simulink model "ModeAdjust"  (R2018b)
settings: Solver=FixedStepDiscrete  StartTime=0.0  StopTime=inf  FixedStep=0.01  RelTol=1e-3
undefined symbols (not defined in the file or in its folder): IfKeSMSbSeatMovBkRclnEnable_Val, IfKeSMSbSeatMovFrwdBkwdEnable_Val, IfKeSMSbSeatMovFtrstEnable_Val, IfKeSMSbSeatMovHdrstFrwdBkwdEnable_Val, IfKeSMSbSeatMovHdUpwdDnwdEnable_Val, IfKeSMSbSeatMovLgrstEnable_Val, IfKeSMSbSeatMovLtwdRtwdEnable_Val, IfVeSMSeStNumConfig, KeSMSbArmscreenMovEnable_Val, KeSMSbSeatMovLgrstExpdEnable_Val, KeSMSuFirstRwStBackPosDelta_Val, KeSMSuFirstRwStBackPosTolr_Val, KeSMSuFirstRwStCushFrntPosDelta_Val, KeSMSuFirstRwStCushFrntPosTolr_Val, KeSMSuFirstRwStCushRePosDelta_Val, KeSMSuFirstRwStCushRePosTolr_Val, KeSMSuFirstRwStFootrestPosDelta_Val, KeSMSuFirstRwStFootrestPosTolr_Val, KeSMSuFirstRwStFwdBkwdPosDelta_Val, KeSMSuFirstRwStFwdBkwdPosTolr_Val, KeSMSuMdMotFinshdTm_Val, KeSMSuMdRetryTm1_Val, KeSMSuModeReqDurgTm_Val, KeSMSuSecRwStArmTochPosDelta_Val, KeSMSuSecRwStArmTochPosTolr_Val, KeSMSuSecRwStBackPosDelta_Val, KeSMSuSecRwStBackPosTolr_Val, KeSMSuSecRwStFtrstUpwdDnwdPosDelta_Val, KeSMSuSecRwStFtrstUpwdDnwdPosTolr_Val, KeSMSuSecRwStFwdBkwdPosDelta_Val, KeSMSuSecRwStFwdBkwdPosTolr_Val, KeSMSuSecRwStHeadrestFwdBkwdPosDelta_Val, KeSMSuSecRwStHeadrestFwdBkwdPosTolr_Val, KeSMSuSecRwStHeadrestUpwdDwnwdPosDelta_Val, KeSMSuSecRwStHeadrestUpwdDwnwdPosTolr_Val, KeSMSuSecRwStLegrestInOutPosDelta_Val, KeSMSuSecRwStLegrestInOutPosTolr_Val, KeSMSuSecRwStLegrestUpwdDwnwdPosDelta_Val, KeSMSuSecRwStLegrestUpwdDwnwdPosTolr_Val, KeSMSuSecRwStLwdRwdPosDelta_Val, KeSMSuSecRwStLwdRwdPosTolr_Val, KeSMSuSecRwStVIPFtrstRefAngle_Val, KeSMSuThirdRwStFwdBkwdPosDelta_Val, KeSMSuThirdRwStFwdBkwdPosTolr_Val, KeSMSuThrdRwCushFoldPosDelta_Val, KeSMSuThrdRwCushFoldPosTolr_Val, KeSMSuThrdRwStBackPosDelta_Val, KeSMSuThrdRwStBackPosTolr_Val, KeSMSw4SLegrstCloseMdSecRwLtStFtrstUpwdDnwdPos_Val, KeSMSw4SLegrstCloseMdSecRwLtStFtrstUpwdDnwdPosMax_Val, KeSMSw4SLegrstCloseMdSecRwLtStFtrstUpwdDnwdPosMin_Val, KeSMSw4SLegrstCloseMdSecRwLtStLgrstOtwdInwdPos_Val, KeSMSw4SLegrstCloseMdSecRwLtStLgrstOtwdInwdPosMax_Val, KeSMSw4SLegrstCloseMdSecRwLtStLgrstOtwdInwdPosMin_Val, KeSMSw4SLegrstCloseMdSecRwLtStLgrstUpwdDnwdPos_Val, KeSMSw4SLegrstCloseMdSecRwLtStLgrstUpwdDnwdPosMax_Val, KeSMSw4SLegrstCloseMdSecRwLtStLgrstUpwdDnwdPosMin_Val, KeSMSw4SLegrstCloseMdSecRwRtStFtrstUpwdDnwdPos_Val, KeSMSw4SLegrstCloseMdSecRwRtStFtrstUpwdDnwdPosMax_Val, KeSMSw4SLegrstCloseMdSecRwRtStFtrstUpwdDnwdPosMin_Val ... (+1138)
libraries: Lib x401
(part 34 of 35)

== stateflow chart ModeAdjust/ModeAdjustRunnable_sys/ModeAdjust/OutNumR3_L ==
  (default) -> (junction 87) : {OutNum =0;}
  (junction 87) -> (junction 69) [order 1] : [HaltReq]
  (junction 87) -> (junction 63) [order 2]
  (junction 69) -> (junction 74)
  (junction 63) -> (junction 72) [order 1] : [EZE]
  (junction 63) -> (junction 80) [order 2]
  (junction 72) -> (junction 77) : {OutNum =1;}
  (junction 80) -> (junction 76) [order 1] : [(VIPL&&is6s7s)]
  (junction 80) -> (junction 52) [order 2]
  (junction 76) -> (junction 56) : {OutNum =2;}
  (junction 52) -> (junction 86) [order 1] : [VIPR&&is7s]
  (junction 52) -> (junction 85) [order 2]
  (junction 86) -> (junction 53) : {OutNum =3;}
  (junction 85) -> (junction 90) [order 1] : [Lug]
  (junction 85) -> (junction 81) [order 2]
  (junction 90) -> (junction 59) : {OutNum =4;}
  (junction 81) -> (junction 92) [order 1] : [FAMLY_R]
  (junction 81) -> (junction 97) [order 2]
  (junction 92) -> (junction 94) : {OutNum =5;}
  (junction 97) -> (junction 99) [order 1] : [FAMLY_L]
  (junction 97) -> (junction 104) [order 2]
  (junction 99) -> (junction 101) : {OutNum =6;}
  (junction 101) -> (junction 104)
  (junction 94) -> (junction 101)
  (junction 59) -> (junction 94)
  (junction 53) -> (junction 59)
  (junction 56) -> (junction 53)
  (junction 77) -> (junction 56)
  (junction 74) -> (junction 77)
  data: HaltReq input boolean; EZE input boolean; VIPL input boolean; VIPR input boolean; Lug input boolean; FAMLY_R input boolean; OutNum output uint8; is7s input boolean; is6s7s input boolean; FAMLY_L input boolean

== stateflow chart ModeAdjust/ModeAdjustRunnable_sys/ModeAdjust/OutNumR2_L ==
  (default) -> (junction 115) : {OutNum =0;}
  (junction 115) -> (junction 117) [order 1] : [HaltReq]
  (junction 115) -> (junction 121) [order 2]
  (junction 117) -> (junction 119)
  (junction 121) -> (junction 123) [order 1] : [EZE]
  (junction 121) -> (junction 127) [order 2]
  (junction 123) -> (junction 125) : {OutNum =1;}
  (junction 127) -> (junction 129) [order 1] : [EZQ]
  (junction 127) -> (junction 133) [order 2]
  (junction 129) -> (junction 131) : {OutNum =2;}
  (junction 133) -> (junction 135) [order 1] : [(VIP&&is6s7s)]
  (junction 133) -> (junction 139) [order 2]
  (junction 135) -> (junction 137) : {OutNum =3;}
  (junction 139) -> (junction 141) [order 1] : [(Recovery&&is6s7s)]
  (junction 139) -> (junction 145) [order 2]
  (junction 141) -> (junction 143) : {OutNum =4;}
  (junction 145) -> (junction 147) [order 1] : [INTM]
  (junction 145) -> (junction 151) [order 2]
  (junction 147) -> (junction 149) : {OutNum =5;}
  (junction 151) -> (junction 153) [order 1] : [FAMLY_L]
  (junction 151) -> (junction 157) [order 2]
  (junction 153) -> (junction 155) : {OutNum =6;}
  (junction 157) -> (junction 159) [order 1] : [FAMLY_R]
  (junction 157) -> (junction 164) [order 2]
  (junction 159) -> (junction 161) : {OutNum =7;}
  (junction 164) -> (junction 166) [order 1] : [LyL]
  (junction 164) -> (junction 177) [order 2]
  (junction 166) -> (junction 168) : {OutNum =8;}
  (junction 177) -> (junction 179) [order 1] : [VIP]
  (junction 177) -> (junction 184) [order 2]
  (junction 179) -> (junction 181) : {OutNum =9;}
  (junction 184) -> (junction 186) [order 1] : [Recovery]
  (junction 184) -> (junction 191) [order 2]
  (junction 186) -> (junction 188) : {OutNum =10;}
  (junction 191) -> (junction 193) [order 1] : [INTMR]
  (junction 191) -> (junction 198) [order 2]
  (junction 193) -> (junction 195) : {OutNum =11;}
  (junction 198) -> (junction 200) [order 1] : [LgrstOpen]
  (junction 198) -> (junction 205) [order 2]
  (junction 200) -> (junction 202) : {OutNum =12;}
  (junction 205) -> (junction 207) [order 1] : [LgrstClose]
  (junction 205) -> (junction 212) [order 2]
  (junction 207) -> (junction 209) : {OutNum =13;}
  (junction 209) -> (junction 212)
  (junction 202) -> (junction 209)
  (junction 195) -> (junction 202)
  (junction 188) -> (junction 195)
  (junction 181) -> (junction 188)
  (junction 168) -> (junction 181)
  (junction 161) -> (junction 168)
  (junction 155) -> (junction 161)
  (junction 149) -> (junction 155)
  (junction 143) -> (junction 149)
  (junction 137) -> (junction 143)
  (junction 131) -> (junction 137)
  (junction 125) -> (junction 131)
  (junction 119) -> (junction 125)
  data: HaltReq input boolean; EZE input boolean; EZQ input boolean; VIP input boolean; Recovery input boolean; OutNum output uint8; INTM input boolean; FAMLY_L input boolean; FAMLY_R input boolean; LyL input boolean; is6s7s input boolean; INTMR input boolean; LgrstOpen input boolean; LgrstClose input boolean

== stateflow chart ModeAdjust/ModeAdjustRunnable_sys/ModeAdjust/LyL/Chart ==
  (default) -> (junction 3) : {
      | failflg =0;
      | }
  (junction 3) -> (junction 5) [order 1] : [!R2Lt_ini]
  (junction 5) -> (junction 9) [order 1] : [R2Lt_done]
  (junction 3) -> (junction 13) [order 2] : {R2Lt_En=false;}
  (junction 5) -> (junction 7) [order 2] : {R2Lt_En=true;}
  (junction 9) -> (junction 11) : {R2Lt_En=false;}
  (junction 7) -> (junction 13)
  (junction 11) -> (junction 7)
  (junction 13) -> (junction 183)
  (junction 183) -> (junction 62)
  (junction 62) -> (junction 76) [order 1] : [!Step1_ini]
  (junction 76) -> (junction 64) [order 1] : [pos<openpos1]
  (junction 64) -> (junction 74) [order 1] : [Step1done]
  (junction 62) -> (junction 68) [order 2] : {
      | StepEn_LgrstStep1=false;
      | }
  (junction 76) -> (junction 105) [order 2]
  (junction 64) -> (junction 66) [order 2] : {
      | StepEn_LgrstStep1=true;
      | StepEn_LgrstStep2=false;
      | StepEn_LgrstStep3=false;
      | }
  (junction 74) -> (junction 102) : {
      | StepEn_LgrstStep1=false;
      | StepEn_LgrstStep2=false;
      | StepEn_LgrstStep3=false;
      | failflg =1;
      | }
  (junction 105) -> (junction 107) [order 1] : [!Step2done||Step1done]
  (junction 105) -> (junction 82) [order 2] : {StepEn_LgrstStep1=true;}
  (junction 107) -> (junction 109) : {StepEn_LgrstStep1=false;}
  (junction 82) -> (junction 68)
  (junction 109) -> (junction 82)
  (junction 102) -> (junction 66)
  (junction 68) -> (junction 85)
  (junction 66) -> (junction 99)
  (junction 85) -> (junction 87) [order 1] : [!Step2_ini]
  (junction 87) -> (junction 94) [order 1] : [Step2done]
  (junction 85) -> (junction 89) [order 2] : {
      | StepEn_LgrstStep2=false;
      | }
  (junction 87) -> (junction 91) [order 2] : {
      | StepEn_LgrstStep2=true;
      | }
  (junction 94) -> (junction 96) : {
      | StepEn_LgrstStep2=false;
      | }
  (junction 91) -> (junction 89)
  (junction 96) -> (junction 91)
  (junction 89) -> (junction 101)
  (junction 101) -> (junction 113) [order 1] : [!Step3_ini]
  (junction 113) -> (junction 115) [order 1] : [(!Step2done)||Step3done]
  (junction 101) -> (junction 118) [order 2] : {
      | StepEn_LgrstStep3=false;
      | }
  (junction 113) -> (junction 116) [order 2] : {
      | StepEn_LgrstStep3=true;
      | }
  (junction 115) -> (junction 122) : {
      | StepEn_LgrstStep3=false;
      | }
  (junction 116) -> (junction 118)
  (junction 122) -> (junction 116)
  (junction 99) -> (junction 122)
  (junction 118) -> (junction 125)
  (junction 125) -> (junction 134) [order 1] : [(Step1done&&Step2done&&Step3done)||failflg]
  (junction 134) -> (junction 136) [order 1] : [chkhdflg]
  (junction 136) -> (junction 168) [order 1] : [HdUp_ini||HdUp_Done]
  (junction 168) -> (junction 173) [order 1] : [HdFwd_ini||HdFwd_Done]
  (junction 125) -> (junction 128) [order 2]
  (junction 134) -> (junction 140) [order 2]
  (junction 136) -> (junction 170) [order 2] : {HdUp_En = true;
      | HdFwd_En =false;}
  (junction 168) -> (junction 178) [order 2] : {HdUp_En = false;
      | HdFwd_En =true;}
  (junction 173) -> (junction 175) : {HdUp_En = false;
      | HdFwd_En =false;}
  (junction 140) -> (junction 142) [order 1] : [HdUp_ini||HdUp_Done]
  (junction 140) -> (junction 151) [order 2] : {HdUp_En = true;}
  (junction 142) -> (junction 149) : {HdUp_En =false;}
  (junction 149) -> (junction 151)
  (junction 151) -> (junction 154)
  (junction 154) -> (junction 156) [order 1] : [HdFwd_ini||HdFwd_Done]
  (junction 154) -> (junction 160) [order 2] : {HdFwd_En =true;}
  (junction 156) -> (junction 158) : {HdFwd_En =false;}
  (junction 158) -> (junction 160)
  (junction 160) -> (junction 163)
  (junction 163) -> (junction 128)
  (junction 170) -> (junction 163)
  (junction 178) -> (junction 170)
  (junction 175) -> (junction 178)
  (junction 128) -> (junction 166)
  data: R2Lt_ini input boolean; R2Lt_done input boolean; R2Lt_En output boolean; pos input uint16; openpos1 input uint16; Step1done input boolean; Step2done input boolean; Step3done input boolean; Step1_ini input boolean; Step2_ini input boolean; Step3_ini input boolean; StepEn_LgrstStep1 output boolean; StepEn_LgrstStep2 output boolean; StepEn_LgrstStep3 output boolean; chkhdflg input boolean; HdUp_Done input boolean; HdFwd_Done input boolean; HdUp_En output boolean; HdFwd_En output boolean; failflg output boolean; HdUp_ini input boolean; HdFwd_ini input boolean

== stateflow chart ModeAdjust/ModeAdjustRunnable_sys/ModeAdjust/OutNumR1_L ==
  (default) -> (junction 78) : {OutNum =0;}
  (junction 78) -> (junction 80) [order 1] : [HaltReq||!is6s7s]
  (junction 78) -> (junction 84) [order 2]
  (junction 80) -> (junction 82)
  (junction 84) -> (junction 86) [order 1] : [EZE]
  (junction 84) -> (junction 91) [order 2]
  (junction 86) -> (junction 88) : {OutNum =1;}
  (junction 91) -> (junction 93) [order 1] : [EZQ]
  (junction 91) -> (junction 98) [order 2]
  (junction 93) -> (junction 95) : {OutNum =2;}
  (junction 98) -> (junction 105)
  (junction 105) -> (junction 107) [order 1] : [Recovery_L]
  (junction 105) -> (junction 112) [order 2]
  (junction 107) -> (junction 109) : {OutNum =3;}
  (junction 112) -> (junction 115) [order 1] : [VIP_L]
  (junction 112) -> (junction 117) [order 2]
  (junction 115) -> (junction 119) : {OutNum =4;}
  (junction 119) -> (junction 117)
  (junction 109) -> (junction 119)
  (junction 95) -> (junction 109)
  (junction 88) -> (junction 95)
  (junction 82) -> (junction 88)
  data: HaltReq input boolean; EZE input boolean; EZQ input boolean; OutNum output uint8; Recovery_L input boolean; VIP_L input boolean; is6s7s input boolean

== stateflow chart ModeAdjust/ModeAdjustRunnable_sys/ModeAdjust/OutNumR1_R ==
  (default) -> (junction 115) : {OutNum =0;}
  (junction 115) -> (junction 97) [order 1] : [HaltReq||!is6s7s]
  (junction 115) -> (junction 91) [order 2]
  (junction 97) -> (junction 102)
  (junction 91) -> (junction 100) [order 1] : [EZE]
  (junction 91) -> (junction 108) [order 2]
  (junction 100) -> (junction 105) : {OutNum =1;}
  (junction 108) -> (junction 104) [order 1] : [EZQ]
  (junction 108) -> (junction 90) [order 2]
  (junction 104) -> (junction 84) : {OutNum =2;}
  (junction 90) -> (junction 80)
  (junction 80) -> (junction 114) [order 1] : [Recovery_R]
  (junction 80) -> (junction 113) [order 2]
  (junction 114) -> (junction 81) : {OutNum =3;}
  (junction 113) -> (junction 118) [order 1] : [VIP_R]
  (junction 113) -> (junction 109) [order 2]
  (junction 118) -> (junction 87) : {OutNum =4;}
  (junction 87) -> (junction 109)
  (junction 81) -> (junction 87)
  (junction 84) -> (junction 81)
  (junction 105) -> (junction 84)
  (junction 102) -> (junction 105)
  data: HaltReq input boolean; EZE input boolean; EZQ input boolean; OutNum output uint8; Recovery_R input boolean; VIP_R input boolean; is6s7s input boolean

== stateflow chart ModeAdjust/ModeAdjustRunnable_sys/ModeAdjust/VIPL4s/Chart ==
  (default) -> (junction 3) : {
      | failflg =0;
      | }
  (junction 3) -> (junction 5) [order 1] : [!R2Lt_ini]
  (junction 5) -> (junction 9) [order 1] : [R2Lt_done]
  (junction 3) -> (junction 13) [order 2] : {R2Lt_En=false;}
  (junction 5) -> (junction 7) [order 2] : {R2Lt_En=true;}
  (junction 9) -> (junction 11) : {R2Lt_En=false;}
  (junction 7) -> (junction 13)
  (junction 11) -> (junction 7)
  (junction 13) -> (junction 183)
  (junction 183) -> (junction 62)
  (junction 62) -> (junction 76) [order 1] : [!Step1_ini]
  (junction 76) -> (junction 64) [order 1] : [pos<openpos1]
  (junction 64) -> (junction 74) [order 1] : [Step1done]
  (junction 62) -> (junction 68) [order 2] : {
      | StepEn_LgrstStep1=false;
      | }
  (junction 76) -> (junction 105) [order 2]
  (junction 64) -> (junction 66) [order 2] : {
      | StepEn_LgrstStep1=true;
      | StepEn_LgrstStep2=false;
      | StepEn_LgrstStep3=false;
      | }
  (junction 74) -> (junction 102) : {
      | StepEn_LgrstStep1=false;
      | StepEn_LgrstStep2=false;
      | StepEn_LgrstStep3=false;
      | failflg =1;
      | }
  (junction 105) -> (junction 107) [order 1] : [!Step2done||Step1done]
  (junction 105) -> (junction 82) [order 2] : {StepEn_LgrstStep1=true;}
  (junction 107) -> (junction 109) : {StepEn_LgrstStep1=false;}
  (junction 82) -> (junction 68)
  (junction 109) -> (junction 82)
  (junction 102) -> (junction 66)
  (junction 68) -> (junction 85)
  (junction 66) -> (junction 99)
  (junction 85) -> (junction 87) [order 1] : [!Step2_ini]
  (junction 87) -> (junction 94) [order 1] : [Step2done]
  (junction 85) -> (junction 89) [order 2] : {
      | StepEn_LgrstStep2=false;
      | }
  (junction 87) -> (junction 91) [order 2] : {
      | StepEn_LgrstStep2=true;
      | }
  (junction 94) -> (junction 96) : {
      | StepEn_LgrstStep2=false;
      | }
  (junction 91) -> (junction 89)
  (junction 96) -> (junction 91)
  (junction 89) -> (junction 101)
  (junction 101) -> (junction 113) [order 1] : [!Step3_ini]
  (junction 113) -> (junction 115) [order 1] : [(!Step2done)||Step3done]
  (junction 101) -> (junction 118) [order 2] : {
      | StepEn_LgrstStep3=false;
      | }
  (junction 113) -> (junction 116) [order 2] : {
      | StepEn_LgrstStep3=true;
      | }
  (junction 115) -> (junction 122) : {
      | StepEn_LgrstStep3=false;
      | }
  (junction 116) -> (junction 118)
  (junction 122) -> (junction 116)
  (junction 99) -> (junction 122)
  (junction 118) -> (junction 125)
  (junction 125) -> (junction 134) [order 1] : [(Step1done&&Step2done&&Step3done)||failflg]
  (junction 134) -> (junction 136) [order 1] : [chkhdflg]
  (junction 136) -> (junction 168) [order 1] : [HdUp_ini||HdUp_Done]
  (junction 168) -> (junction 173) [order 1] : [HdFwd_ini||HdFwd_Done]
  (junction 125) -> (junction 128) [order 2]
  (junction 134) -> (junction 140) [order 2]
  (junction 136) -> (junction 170) [order 2] : {HdUp_En = true;
      | HdFwd_En =false;}
  (junction 168) -> (junction 178) [order 2] : {HdUp_En = false;
      | HdFwd_En =true;}
  (junction 173) -> (junction 175) : {HdUp_En = false;
      | HdFwd_En =false;}
  (junction 140) -> (junction 142) [order 1] : [HdUp_ini||HdUp_Done]
  (junction 140) -> (junction 151) [order 2] : {HdUp_En = true;}
  (junction 142) -> (junction 149) : {HdUp_En =false;}
  (junction 149) -> (junction 151)
  (junction 151) -> (junction 154)
  (junction 154) -> (junction 156) [order 1] : [HdFwd_ini||HdFwd_Done]
  (junction 154) -> (junction 160) [order 2] : {HdFwd_En =true;}
  (junction 156) -> (junction 158) : {HdFwd_En =false;}
  (junction 158) -> (junction 160)
  (junction 160) -> (junction 163)
  (junction 163) -> (junction 128)
  (junction 170) -> (junction 163)
  (junction 178) -> (junction 170)
  (junction 175) -> (junction 178)
  (junction 128) -> (junction 166)
  data: R2Lt_ini input boolean; R2Lt_done input boolean; R2Lt_En output boolean; pos input uint16; openpos1 input uint16; Step1done input boolean; Step2done input boolean; Step3done input boolean; Step1_ini input boolean; Step2_ini input boolean; Step3_ini input boolean; StepEn_LgrstStep1 output boolean; StepEn_LgrstStep2 output boolean; StepEn_LgrstStep3 output boolean; chkhdflg input boolean; HdUp_Done input boolean; HdFwd_Done input boolean; HdUp_En output boolean; HdFwd_En output boolean; failflg output boolean; HdUp_ini input boolean; HdFwd_ini input boolean

== stateflow chart ModeAdjust/ModeAdjustRunnable_sys/ModeAdjust/ModeEnChek/Chart3 ==
  (default) -> (junction 3)
  (junction 3) -> (junction 9) : {i = 0;}
  (junction 9) -> (junction 4) [order 1] : [i < 32]
  (junction 4) -> (junction 1) : {
      | temp_var = 0x00000001 & (ModeState32>>i);
      | ModeArray[i] =boolean(temp_var);
      | }
  (junction 1) -> (junction 9) : {i++;}
  (junction 9) -> (junction 5) [order 2]
  data: temp_var local uint32; ModeState32 input uint32; ModeArray output boolean size=32; i local uint8

== stateflow chart ModeAdjust/ModeAdjustRunnable_sys/ModeAdjust/FAMLYL/Chart1 ==
  (default) -> (junction 51)
  (junction 51) -> (junction 53) [order 1] : [LeftDone]
  (junction 51) -> (junction 7) [order 2] : {
      | IfVeSMSbSecRwRtStRclCmdSrv_Val_write=IfVeSMSbSecRwRtStRclCmdSrv_Val_writeRaw;
      | IfVeSMSbThdRwRtStRclCmdSrv_Val_write=IfVeSMSbThdRwRtStRclCmdSrv_Val_writeRaw;
      | IfVeSMSuSecRwLtStRclCmdSrv_Val_write=IfVeSMSuSecRwLtStRclCmdSrv_Val_writeRaw;
      | IfVeSMSbThdRwLtStRclCmdSrv_Val_write=IfVeSMSbThdRwLtStRclCmdSrv_Val_writeRaw;
      | Md_L_DoneOk=false;
      | Md_L_DoneFailed=false;
      | }
  (junction 53) -> (junction 55) : {
      | IfVeSMSbSecRwRtStRclCmdSrv_Val_write=false;
      | IfVeSMSbThdRwRtStRclCmdSrv_Val_write=false;
      | IfVeSMSuSecRwLtStRclCmdSrv_Val_write=false;
      | IfVeSMSbThdRwLtStRclCmdSrv_Val_write=false;
      | Md_L_DoneOk=Md_L_DoneOkRaw;
      | Md_L_DoneFailed=Md_L_DoneFailedRaw;
      | }
  (junction 55) -> (junction 7)
  (junction 7) -> (junction 46)
  data: LeftDone input boolean; IfVeSMSbSecRwRtStRclCmdSrv_Val_write output boolean; IfVeSMSuSecRwLtStRclCmdSrv_Val_write output boolean; IfVeSMSbSecRwRtStRclCmdSrv_Val_writeRaw input; IfVeSMSuSecRwLtStRclCmdSrv_Val_writeRaw input; Md_L_DoneOkRaw input; Md_L_DoneFailedRaw input; Md_L_DoneOk output boolean; Md_L_DoneFailed output boolean; IfVeSMSbThdRwRtStRclCmdSrv_Val_writeRaw input; IfVeSMSbThdRwRtStRclCmdSrv_Val_write output boolean; IfVeSMSbThdRwLtStRclCmdSrv_Val_writeRaw input; IfVeSMSbThdRwLtStRclCmdSrv_Val_write output boolean

== stateflow chart ModeAdjust/ModeAdjustRunnable_sys/ModeAdjust/FAMLYL/Chart2 ==
  (default) -> (junction 487)
  (junction 487) -> (junction 489) [order 1] : [!L_R2Step2_ini]
  (junction 489) -> (junction 488) [order 1] : [L_R2_Step2done]
  (junction 487) -> (junction 483) [order 2] : {L_R2Step2=false;}
  (junction 489) -> (junction 484) [order 2] : {L_R2Step2=true;}
  (junction 488) -> (junction 490) : {L_R2Step2=false;}
  (junction 484) -> (junction 483)
  (junction 490) -> (junction 484)
  (junction 483) -> (junction 460)
  (junction 460) -> (junction 458) [order 1] : [!R_R2Step2_ini]
  (junction 458) -> (junction 463) [order 1] : [R_R2_Step2done]
  (junction 460) -> (junction 466) [order 2] : {R_R2Step2=false;}
  (junction 458) -> (junction 464) [order 2] : {R_R2Step2=true;}
  (junction 463) -> (junction 465) : {R_R2Step2=false;}
  (junction 464) -> (junction 466)
  (junction 465) -> (junction 464)
  (junction 466) -> (junction 461)
  (junction 461) -> (junction 467) [order 1] : [!R_R3_Step1_ini]
  (junction 467) -> (junction 459) [order 1] : [R_R3_Step1done]
  (junction 461) -> (junction 457) [order 2] : {R_R3Step1=false;}
  (junction 467) -> (junction 462) [order 2] : {R_R3Step1=true;}
  (junction 459) -> (junction 455) : {R_R3Step1=false;}
  (junction 462) -> (junction 457)
  (junction 455) -> (junction 462)
  (junction 457) -> (junction 498)
  (junction 498) -> (junction 499) [order 1] : [!L_R3_Step1_ini]
  (junction 499) -> (junction 500) [order 1] : [L_R3_Step1done]
  (junction 498) -> (junction 510) [order 2] : {L_R3Step1=false;}
  (junction 499) -> (junction 508) [order 2] : {L_R3Step1=true;}
  (junction 500) -> (junction 512) : {L_R3Step1=false;}
  (junction 508) -> (junction 510)
  (junction 512) -> (junction 508)
  (junction 510) -> (junction 513)
  data: R_R3Step1 output boolean; R_R2Step2 output boolean; L_R2Step2 output boolean; R_R2Step2_ini input boolean; L_R2Step2_ini input boolean; R_R2_Step2done input boolean; L_R2_Step2done input boolean; R_R3_Step1_ini input boolean; R_R3_Step1done input boolean; L_R3Step1 output boolean; L_R3_Step1_ini input boolean; L_R3_Step1done input boolean

== stateflow chart ModeAdjust/ModeAdjustRunnable_sys/ModeAdjust/FAMLYR/Chart1 ==
  (default) -> (junction 51)
  (junction 51) -> (junction 53) [order 1] : [LeftDone]
  (junction 51) -> (junction 7) [order 2] : {
      | IfVeSMSbSecRwRtStRclCmdSrv_Val_write=IfVeSMSbSecRwRtStRclCmdSrv_Val_writeRaw;
      | IfVeSMSbThdRwRtStRclCmdSrv_Val_write=IfVeSMSbThdRwRtStRclCmdSrv_Val_writeRaw;
      | IfVeSMSuSecRwLtStRclCmdSrv_Val_write=IfVeSMSuSecRwLtStRclCmdSrv_Val_writeRaw;
      | IfVeSMSbThdRwLtStRclCmdSrv_Val_write=IfVeSMSbThdRwLtStRclCmdSrv_Val_writeRaw;
      | Md_L_DoneOk=false;
      | Md_L_DoneFailed=false;
      | }
  (junction 53) -> (junction 55) : {
      | IfVeSMSbSecRwRtStRclCmdSrv_Val_write=false;
      | IfVeSMSbThdRwRtStRclCmdSrv_Val_write=false;
      | IfVeSMSuSecRwLtStRclCmdSrv_Val_write=false;
      | IfVeSMSbThdRwLtStRclCmdSrv_Val_write=false;
      | Md_L_DoneOk=Md_L_DoneOkRaw;
      | Md_L_DoneFailed=Md_L_DoneFailedRaw;
      | }
  (junction 55) -> (junction 7)
  (junction 7) -> (junction 46)
  data: LeftDone input boolean; IfVeSMSbSecRwRtStRclCmdSrv_Val_write output boolean; IfVeSMSuSecRwLtStRclCmdSrv_Val_write output boolean; IfVeSMSbSecRwRtStRclCmdSrv_Val_writeRaw input; IfVeSMSuSecRwLtStRclCmdSrv_Val_writeRaw input; Md_L_DoneOkRaw input; Md_L_DoneFailedRaw input; Md_L_DoneOk output boolean; Md_L_DoneFailed output boolean; IfVeSMSbThdRwRtStRclCmdSrv_Val_writeRaw input; IfVeSMSbThdRwRtStRclCmdSrv_Val_write output boolean; IfVeSMSbThdRwLtStRclCmdSrv_Val_writeRaw input; IfVeSMSbThdRwLtStRclCmdSrv_Val_write output boolean

== stateflow chart ModeAdjust/ModeAdjustRunnable_sys/ModeAdjust/FAMLYR/Chart2 ==
  (default) -> (junction 487)
  (junction 487) -> (junction 489) [order 1] : [!L_R2Step2_ini]
  (junction 489) -> (junction 488) [order 1] : [L_R2_Step2done]
  (junction 487) -> (junction 483) [order 2] : {L_R2Step2=false;}
  (junction 489) -> (junction 484) [order 2] : {L_R2Step2=true;}
  (junction 488) -> (junction 490) : {L_R2Step2=false;}
  (junction 484) -> (junction 483)
  (junction 490) -> (junction 484)
  (junction 483) -> (junction 460)
  (junction 460) -> (junction 458) [order 1] : [!R_R2Step2_ini]
  (junction 458) -> (junction 463) [order 1] : [R_R2_Step2done]
  (junction 460) -> (junction 466) [order 2] : {R_R2Step2=false;}
  (junction 458) -> (junction 464) [order 2] : {R_R2Step2=true;}
  (junction 463) -> (junction 465) : {R_R2Step2=false;}
  (junction 464) -> (junction 466)
  (junction 465) -> (junction 464)
  (junction 466) -> (junction 461)
  (junction 461) -> (junction 467) [order 1] : [!R_R3_Step1_ini]
  (junction 467) -> (junction 459) [order 1] : [R_R3_Step1done]
  (junction 461) -> (junction 457) [order 2] : {R_R3Step1=false;}
  (junction 467) -> (junction 462) [order 2] : {R_R3Step1=true;}
  (junction 459) -> (junction 455) : {R_R3Step1=false;}
  (junction 462) -> (junction 457)
  (junction 455) -> (junction 462)
  (junction 457) -> (junction 511)
  (junction 511) -> (junction 498) [order 1] : [!L_R3_Step1_ini]
  (junction 498) -> (junction 501) [order 1] : [L_R3_Step1done]
  (junction 511) -> (junction 506) [order 2] : {L_R3Step1=false;}
  (junction 498) -> (junction 509) [order 2] : {L_R3Step1=true;}
  (junction 501) -> (junction 505) : {L_R3Step1=false;}
  (junction 509) -> (junction 506)
  (junction 505) -> (junction 509)
  (junction 506) -> (junction 454)
  data: R_R3Step1 output boolean; R_R2Step2 output boolean; L_R2Step2 output boolean; R_R2Step2_ini input boolean; L_R2Step2_ini input boolean; R_R2_Step2done input boolean; L_R2_Step2done input boolean; R_R3_Step1_ini input boolean; R_R3_Step1done input boolean; L_R3Step1 output boolean; L_R3_Step1_ini input boolean; L_R3_Step1done input boolean

== stateflow chart ModeAdjust/ModeAdjustRunnable_sys/ModeAdjust/INTML/Chart ==
  (default) -> (junction 10)
  (junction 10) -> (junction 58) [order 1] : [!L_R2_ini]
  (junction 58) -> (junction 25) [order 1] : [L_R2_done]
  (junction 10) -> (junction 26) [order 2] : {L_R2_en=false;}
  (junction 58) -> (junction 35) [order 2] : {L_R2_en=true;}
  (junction 25) -> (junction 18) : {
      | L_R2_en=false;
      | }
  (junction 35) -> (junction 26)
  (junction 18) -> (junction 35)
  (junction 26) -> (junction 129)
  (junction 129) -> (junction 133) [order 1] : [!R_R2_ini]
  (junction 133) -> (junction 128) [order 1] : [R_R2_done]
  (junction 129) -> (junction 131) [order 2] : {R_R2_en=false;}
  (junction 133) -> (junction 127) [order 2] : {R_R2_en=true;}
  (junction 128) -> (junction 125) : {
      | R_R2_en=false;
      | }
  (junction 127) -> (junction 131)
  (junction 125) -> (junction 127)
  (junction 131) -> (junction 134)
  data: L_R2_ini input boolean; L_R2_done input boolean; R_R2_en output boolean; L_R2_en output boolean; R_R2_ini input boolean; R_R2_done input boolean

== stateflow chart ModeAdjust/ModeAdjustRunnable_sys/ModeAdjust/INTML/Chart1 ==
  (default) -> (junction 1)
  (junction 1) -> (junction 3) [order 1] : [StepAlldone]
  (junction 1) -> (junction 7) [order 2] : {
      | IfVeSMSbSecRwRtStRclCmdSrv_Val_write=IfVeSMSbSecRwRtStRclCmdSrv_Val_writeRaw;
      | IfVeSMSuSecRwLtStRclCmdSrv_Val_write=IfVeSMSuSecRwLtStRclCmdSrv_Val_writeRaw;
      | isINTMDoneOk=false;
      | isINTMDoneFailed=false;
      | }
  (junction 3) -> (junction 5) : {
      | IfVeSMSbSecRwRtStRclCmdSrv_Val_write=false;
      | IfVeSMSuSecRwLtStRclCmdSrv_Val_write=false;
      | isINTMDoneOk=isINTMDoneOkRaw;
      | isINTMDoneFailed=isINTMDoneFailedRaw;
      | }
  (junction 5) -> (junction 7)
  (junction 7) -> (junction 10)
  data: StepAlldone input boolean; IfVeSMSbSecRwRtStRclCmdSrv_Val_write output boolean; IfVeSMSuSecRwLtStRclCmdSrv_Val_write output boolean; isINTMDoneOk output boolean; isINTMDoneFailed output boolean; IfVeSMSbSecRwRtStRclCmdSrv_Val_writeRaw input; IfVeSMSuSecRwLtStRclCmdSrv_Val_writeRaw input; isINTMDoneFailedRaw input; isINTMDoneOkRaw input

== stateflow chart ModeAdjust/ModeAdjustRunnable_sys/ModeAdjust/OutNumR2_R ==
  (default) -> (junction 132) : {OutNum =0;}
  (junction 132) -> (junction 136) [order 1] : [HaltReq]
  (junction 132) -> (junction 134) [order 2]
  (junction 136) -> (junction 183)
  (junction 134) -> (junction 138) [order 1] : [EZE]
  (junction 134) -> (junction 145) [order 2]
  (junction 138) -> (junction 140) : {OutNum =1;}
  (junction 145) -> (junction 147) [order 1] : [EZQ]
  (junction 145) -> (junction 154) [order 2]
  (junction 147) -> (junction 149) : {OutNum =2;}
  (junction 154) -> (junction 156) [order 1] : [(VIP&&is6s7s)]
  (junction 154) -> (junction 163) [order 2]
  (junction 156) -> (junction 158) : {OutNum =3;}
  (junction 163) -> (junction 165) [order 1] : [(Recovery&&is6s7s)]
  (junction 163) -> (junction 172) [order 2]
  (junction 165) -> (junction 167) : {OutNum =4;}
  (junction 172) -> (junction 174) [order 1] : [INTM]
  (junction 172) -> (junction 193) [order 2]
  (junction 174) -> (junction 176) : {OutNum =5;}
  (junction 193) -> (junction 195) [order 1] : [FAMLY_L]
  (junction 193) -> (junction 199) [order 2]
  (junction 195) -> (junction 197) : {OutNum =6;}
  (junction 199) -> (junction 201) [order 1] : [FAMLY_R]
  (junction 199) -> (junction 208) [order 2]
  (junction 201) -> (junction 203) : {OutNum =7;}
  (junction 208) -> (junction 210) [order 1] : [LyR]
  (junction 208) -> (junction 215) [order 2]
  (junction 210) -> (junction 212) : {OutNum =8;}
  (junction 215) -> (junction 217) [order 1] : [VIP]
  (junction 215) -> (junction 223) [order 2]
  (junction 217) -> (junction 219) : {OutNum =9;}
  (junction 223) -> (junction 225) [order 1] : [Recovery]
  (junction 223) -> (junction 230) [order 2]
  (junction 225) -> (junction 227) : {OutNum =10;}
  (junction 230) -> (junction 232) [order 1] : [INTMR]
  (junction 230) -> (junction 237) [order 2]
  (junction 232) -> (junction 234) : {OutNum =11;}
  (junction 237) -> (junction 239) [order 1] : [LgrstOpen]
  (junction 237) -> (junction 244) [order 2]
  (junction 239) -> (junction 241) : {OutNum =12;}
  (junction 244) -> (junction 246) [order 1] : [LgrstClose]
  (junction 244) -> (junction 251) [order 2]
  (junction 246) -> (junction 248) : {OutNum =13;}
  (junction 248) -> (junction 251)
  (junction 241) -> (junction 248)
  (junction 234) -> (junction 241)
  (junction 227) -> (junction 234)
  (junction 219) -> (junction 227)
  (junction 212) -> (junction 219)
  (junction 203) -> (junction 212)
  (junction 197) -> (junction 203)
  (junction 176) -> (junction 197)
  (junction 167) -> (junction 176)
  (junction 158) -> (junction 167)
  (junction 149) -> (junction 158)
  (junction 140) -> (junction 149)
  (junction 183) -> (junction 140)
  data: HaltReq input boolean; EZE input boolean; EZQ input boolean; VIP input boolean; Recovery input boolean; OutNum output uint8; INTM input boolean; FAMLY_L input boolean; FAMLY_R input boolean; LyR input boolean; is6s7s input boolean; INTMR input boolean; LgrstOpen input boolean; LgrstClose input boolean

== stateflow chart ModeAdjust/ModeAdjustRunnable_sys/ModeAdjust/LyL/Chart1 ==
  (default) -> (junction 1)
  (junction 1) -> (junction 3) [order 1] : [Left_Done]
  (junction 1) -> (junction 7) [order 2] : {
      | IfVeSMSuSecRwLtStRclCmdSrv_Val_write=IfVeSMSuSecRwLtStRclCmdSrv_Val_writeRaw;
      | Md_L_DoneOk=false;
      | Md_L_DoneFailed=false;
      | }
  (junction 3) -> (junction 5) : {
      | IfVeSMSuSecRwLtStRclCmdSrv_Val_write=false;
      | Md_L_DoneOk=Md_L_DoneOkRaw;
      | Md_L_DoneFailed=Md_L_DoneFailedRaw;
      | }
  (junction 5) -> (junction 7)
  (junction 7) -> (junction 10)
  data: Left_Done input boolean; IfVeSMSuSecRwLtStRclCmdSrv_Val_write output boolean; IfVeSMSuSecRwLtStRclCmdSrv_Val_writeRaw input; Md_L_DoneOkRaw input; Md_L_DoneFailedRaw input; Md_L_DoneOk output boolean; Md_L_DoneFailed output boolean

== stateflow chart ModeAdjust/ModeAdjustRunnable_sys/ModeAdjust/LyR/Chart ==
  (default) -> (junction 3) : {
      | failflg =0;
      | }
  (junction 3) -> (junction 5) [order 1] : [!R2Lt_ini]
  (junction 5) -> (junction 9) [order 1] : [R2Lt_done]
  (junction 3) -> (junction 13) [order 2] : {R2Lt_En=false;}
  (junction 5) -> (junction 7) [order 2] : {R2Lt_En=true;}
  (junction 9) -> (junction 11) : {R2Lt_En=false;}
  (junction 7) -> (junction 13)
  (junction 11) -> (junction 7)
  (junction 13) -> (junction 183)
  (junction 183) -> (junction 62)
  (junction 62) -> (junction 76) [order 1] : [!Step1_ini]
  (junction 76) -> (junction 64) [order 1] : [pos<openpos1]
  (junction 64) -> (junction 74) [order 1] : [Step1done]
  (junction 62) -> (junction 68) [order 2] : {
      | StepEn_LgrstStep1=false;
      | }
  (junction 76) -> (junction 105) [order 2]
  (junction 64) -> (junction 66) [order 2] : {
      | StepEn_LgrstStep1=true;
      | StepEn_LgrstStep2=false;
      | StepEn_LgrstStep3=false;
      | }
  (junction 74) -> (junction 102) : {
      | StepEn_LgrstStep1=false;
      | StepEn_LgrstStep2=false;
      | StepEn_LgrstStep3=false;
      | failflg =1;
      | }
  (junction 105) -> (junction 107) [order 1] : [!Step2done||Step1done]
  (junction 105) -> (junction 82) [order 2] : {StepEn_LgrstStep1=true;}
  (junction 107) -> (junction 109) : {StepEn_LgrstStep1=false;}
  (junction 82) -> (junction 68)
  (junction 109) -> (junction 82)
  (junction 102) -> (junction 66)
  (junction 68) -> (junction 85)
  (junction 66) -> (junction 99)
  (junction 85) -> (junction 87) [order 1] : [!Step2_ini]
  (junction 87) -> (junction 94) [order 1] : [Step2done]
  (junction 85) -> (junction 89) [order 2] : {
      | StepEn_LgrstStep2=false;
      | }
  (junction 87) -> (junction 91) [order 2] : {
      | StepEn_LgrstStep2=true;
      | }
  (junction 94) -> (junction 96) : {
      | StepEn_LgrstStep2=false;
      | }
  (junction 91) -> (junction 89)
  (junction 96) -> (junction 91)
  (junction 89) -> (junction 101)
  (junction 101) -> (junction 113) [order 1] : [!Step3_ini]
  (junction 113) -> (junction 115) [order 1] : [(!Step2done)||Step3done]
  (junction 101) -> (junction 118) [order 2] : {
      | StepEn_LgrstStep3=false;
      | }
  (junction 113) -> (junction 116) [order 2] : {
      | StepEn_LgrstStep3=true;
      | }
  (junction 115) -> (junction 122) : {
      | StepEn_LgrstStep3=false;
      | }
  (junction 116) -> (junction 118)
  (junction 122) -> (junction 116)
  (junction 99) -> (junction 122)
  (junction 118) -> (junction 125)
  (junction 125) -> (junction 134) [order 1] : [(Step1done&&Step2done&&Step3done)||failflg]
  (junction 134) -> (junction 136) [order 1] : [chkhdflg]
  (junction 136) -> (junction 168) [order 1] : [HdUp_ini||HdUp_Done]
  (junction 168) -> (junction 173) [order 1] : [HdFwd_ini||HdFwd_Done]
  (junction 125) -> (junction 128) [order 2]
  (junction 134) -> (junction 140) [order 2]
  (junction 136) -> (junction 170) [order 2] : {HdUp_En = true;
      | HdFwd_En =false;}
  (junction 168) -> (junction 178) [order 2] : {HdUp_En = false;
      | HdFwd_En =true;}
  (junction 173) -> (junction 175) : {HdUp_En = false;
      | HdFwd_En =false;}
  (junction 140) -> (junction 142) [order 1] : [HdUp_ini||HdUp_Done]
  (junction 140) -> (junction 151) [order 2] : {HdUp_En = true;}
  (junction 142) -> (junction 149) : {HdUp_En =false;}
  (junction 149) -> (junction 151)
  (junction 151) -> (junction 154)
  (junction 154) -> (junction 156) [order 1] : [HdFwd_ini||HdFwd_Done]
  (junction 154) -> (junction 160) [order 2] : {HdFwd_En =true;}
  (junction 156) -> (junction 158) : {HdFwd_En =false;}
  (junction 158) -> (junction 160)
  (junction 160) -> (junction 163)
  (junction 163) -> (junction 128)
  (junction 170) -> (junction 163)
  (junction 178) -> (junction 170)
  (junction 175) -> (junction 178)
  (junction 128) -> (junction 166)
  data: R2Lt_ini input boolean; R2Lt_done input boolean; R2Lt_En output boolean; pos input uint16; openpos1 input uint16; Step1done input boolean; Step2done input boolean; Step3done input boolean; Step1_ini input boolean; Step2_ini input boolean; Step3_ini input boolean; StepEn_LgrstStep1 output boolean; StepEn_LgrstStep2 output boolean; StepEn_LgrstStep3 output boolean; chkhdflg input boolean; HdUp_Done input boolean; HdFwd_Done input boolean; HdUp_En output boolean; HdFwd_En output boolean; failflg output boolean; HdUp_ini input boolean; HdFwd_ini input boolean

== stateflow chart ModeAdjust/ModeAdjustRunnable_sys/ModeAdjust/LyR/Chart1 ==
  (default) -> (junction 1)
  (junction 1) -> (junction 3) [order 1] : [Left_Done]
  (junction 1) -> (junction 7) [order 2] : {
      | IfVeSMSuSecRwLtStRclCmdSrv_Val_write=IfVeSMSuSecRwLtStRclCmdSrv_Val_writeRaw;
      | Md_L_DoneOk=false;
      | Md_L_DoneFailed=false;
      | }
  (junction 3) -> (junction 5) : {
      | IfVeSMSuSecRwLtStRclCmdSrv_Val_write=false;
      | Md_L_DoneOk=Md_L_DoneOkRaw;
      | Md_L_DoneFailed=Md_L_DoneFailedRaw;
      | }
  (junction 5) -> (junction 7)
  (junction 7) -> (junction 10)
  data: Left_Done input boolean; IfVeSMSuSecRwLtStRclCmdSrv_Val_write output boolean; IfVeSMSuSecRwLtStRclCmdSrv_Val_writeRaw input; Md_L_DoneOkRaw input; Md_L_DoneFailedRaw input; Md_L_DoneOk output boolean; Md_L_DoneFailed output boolean

== stateflow chart ModeAdjust/ModeAdjustRunnable_sys/ModeAdjust/VIPR4s/Chart ==
  (default) -> (junction 3) : {
      | failflg =0;
      | }
  (junction 3) -> (junction 5) [order 1] : [!R2Lt_ini]
  (junction 5) -> (junction 9) [order 1] : [R2Lt_done]
  (junction 3) -> (junction 13) [order 2] : {R2Lt_En=false;}
  (junction 5) -> (junction 7) [order 2] : {R2Lt_En=true;}
  (junction 9) -> (junction 11) : {R2Lt_En=false;}
  (junction 7) -> (junction 13)
  (junction 11) -> (junction 7)
  (junction 13) -> (junction 183)
  (junction 183) -> (junction 62)
  (junction 62) -> (junction 76) [order 1] : [!Step1_ini]
  (junction 76) -> (junction 64) [order 1] : [pos<openpos1]
  (junction 64) -> (junction 74) [order 1] : [Step1done]
  (junction 62) -> (junction 68) [order 2] : {
      | StepEn_LgrstStep1=false;
      | }
  (junction 76) -> (junction 105) [order 2]
  (junction 64) -> (junction 66) [order 2] : {
      | StepEn_LgrstStep1=true;
      | StepEn_LgrstStep2=false;
      | StepEn_LgrstStep3=false;
      | }
  (junction 74) -> (junction 102) : {
      | StepEn_LgrstStep1=false;
      | StepEn_LgrstStep2=false;
      | StepEn_LgrstStep3=false;
      | failflg =1;
      | }
  (junction 105) -> (junction 107) [order 1] : [!Step2done||Step1done]
  (junction 105) -> (junction 82) [order 2] : {StepEn_LgrstStep1=true;}
  (junction 107) -> (junction 109) : {StepEn_LgrstStep1=false;}
  (junction 82) -> (junction 68)
  (junction 109) -> (junction 82)
  (junction 102) -> (junction 66)
  (junction 68) -> (junction 85)
  (junction 66) -> (junction 99)
  (junction 85) -> (junction 87) [order 1] : [!Step2_ini]
  (junction 87) -> (junction 94) [order 1] : [Step2done]
  (junction 85) -> (junction 89) [order 2] : {
      | StepEn_LgrstStep2=false;
      | }
  (junction 87) -> (junction 91) [order 2] : {
      | StepEn_LgrstStep2=true;
      | }
  (junction 94) -> (junction 96) : {
      | StepEn_LgrstStep2=false;
      | }
  (junction 91) -> (junction 89)
  (junction 96) -> (junction 91)
  (junction 89) -> (junction 101)
  (junction 101) -> (junction 113) [order 1] : [!Step3_ini]
  (junction 113) -> (junction 115) [order 1] : [(!Step2done)||Step3done]
  (junction 101) -> (junction 118) [order 2] : {
      | StepEn_LgrstStep3=false;
      | }
  (junction 113) -> (junction 116) [order 2] : {
      | StepEn_LgrstStep3=true;
      | }
  (junction 115) -> (junction 122) : {
      | StepEn_LgrstStep3=false;
      | }
  (junction 116) -> (junction 118)
  (junction 122) -> (junction 116)
  (junction 99) -> (junction 122)
  (junction 118) -> (junction 125)
  (junction 125) -> (junction 134) [order 1] : [(Step1done&&Step2done&&Step3done)||failflg]
  (junction 134) -> (junction 136) [order 1] : [chkhdflg]
  (junction 136) -> (junction 168) [order 1] : [HdUp_ini||HdUp_Done]
  (junction 168) -> (junction 173) [order 1] : [HdFwd_ini||HdFwd_Done]
  (junction 125) -> (junction 128) [order 2]
  (junction 134) -> (junction 140) [order 2]
  (junction 136) -> (junction 170) [order 2] : {HdUp_En = true;
      | HdFwd_En =false;}
  (junction 168) -> (junction 178) [order 2] : {HdUp_En = false;
      | HdFwd_En =true;}
  (junction 173) -> (junction 175) : {HdUp_En = false;
      | HdFwd_En =false;}
  (junction 140) -> (junction 142) [order 1] : [HdUp_ini||HdUp_Done]
  (junction 140) -> (junction 151) [order 2] : {HdUp_En = true;}
  (junction 142) -> (junction 149) : {HdUp_En =false;}
  (junction 149) -> (junction 151)
  (junction 151) -> (junction 154)
  (junction 154) -> (junction 156) [order 1] : [HdFwd_ini||HdFwd_Done]
  (junction 154) -> (junction 160) [order 2] : {HdFwd_En =true;}
  (junction 156) -> (junction 158) : {HdFwd_En =false;}
  (junction 158) -> (junction 160)
  (junction 160) -> (junction 163)
  (junction 163) -> (junction 128)
  (junction 170) -> (junction 163)
  (junction 178) -> (junction 170)
  (junction 175) -> (junction 178)
  (junction 128) -> (junction 166)
  data: R2Lt_ini input boolean; R2Lt_done input boolean; R2Lt_En output boolean; pos input uint16; openpos1 input uint16; Step1done input boolean; Step2done input boolean; Step3done input boolean; Step1_ini input boolean; Step2_ini input boolean; Step3_ini input boolean; StepEn_LgrstStep1 output boolean; StepEn_LgrstStep2 output boolean; StepEn_LgrstStep3 output boolean; chkhdflg input boolean; HdUp_Done input boolean; HdFwd_Done input boolean; HdUp_En output boolean; HdFwd_En output boolean; failflg output boolean; HdUp_ini input boolean; HdFwd_ini input boolean

== stateflow chart ModeAdjust/ModeAdjustRunnable_sys/ModeAdjust/VIPL4s/Chart1 ==
  (default) -> (junction 1)
  (junction 1) -> (junction 3) [order 1] : [Left_Done]
  (junction 1) -> (junction 7) [order 2] : {
      | IfVeSMSuSecRwLtStRclCmdSrv_Val_write=IfVeSMSuSecRwLtStRclCmdSrv_Val_writeRaw;
      | Md_L_DoneOk=false;
      | Md_L_DoneFailed=false;
      | }
  (junction 3) -> (junction 5) : {
      | IfVeSMSuSecRwLtStRclCmdSrv_Val_write=false;
      | Md_L_DoneOk=Md_L_DoneOkRaw;
      | Md_L_DoneFailed=Md_L_DoneFailedRaw;
      | }
  (junction 5) -> (junction 7)
  (junction 7) -> (junction 10)
  data: Left_Done input boolean; IfVeSMSuSecRwLtStRclCmdSrv_Val_write output boolean; IfVeSMSuSecRwLtStRclCmdSrv_Val_writeRaw input; Md_L_DoneOkRaw input; Md_L_DoneFailedRaw input; Md_L_DoneOk output boolean; Md_L_DoneFailed output boolean

== stateflow chart ModeAdjust/ModeAdjustRunnable_sys/ModeAdjust/ArrivedAtTargetPosChk/VIP/Pass/FtTargtCal ==
  (default) -> (junction 4)
  (junction 4) -> (junction 6) : {
      | FtTargetAngle = KeSMSuSecRwStVIPFtrstRefAngle-BkReclnUpwdDnwdPos/4000*78;
      | }
  (junction 6) -> (junction 9) [order 1] : [FtTargetAngle<0]
  (junction 6) -> (junction 13) [order 2]
  (junction 9) -> (junction 11) : {
      | FtTargetAngle=0;
      | }
  (junction 11) -> (junction 13)
  (junction 13) -> (junction 16)
  (junction 16) -> (junction 18) [order 1] : [FtTargetAngle>=108.2216]
  (junction 16) -> (junction 25) [order 2] : {
      | n=(sqrt(26933.84-(cos(FtTargetAngle*3.14159/180+0.43)*8110))-139.91)/0.12;
      | }
  (junction 18) -> (junction 20) : {
      | FtTargetPos=4000;
      | }
  (junction 25) -> (junction 28) : {
      | tmpTargetPos = n*4000;
      | tmpTargetPos = tmpTargetPos/335.245;
      | FtTargetPos = tmpTargetPos;
      | }
  (junction 20) -> (junction 28)
  (junction 28) -> (junction 32)
  data: BkReclnUpwdDnwdPos input single; KeSMSuSecRwStVIPFtrstRefAngle input single; FtTargetPos output uint16; FtTargetAngle local single; n local single; tmpTargetPos local single

== stateflow chart ModeAdjust/ModeAdjustRunnable_sys/ModeAdjust/VIPR4s/Chart1 ==
  (default) -> (junction 1)
  (junction 1) -> (junction 3) [order 1] : [Left_Done]
  (junction 1) -> (junction 7) [order 2] : {
      | IfVeSMSuSecRwLtStRclCmdSrv_Val_write=IfVeSMSuSecRwLtStRclCmdSrv_Val_writeRaw;
      | Md_L_DoneOk=false;
      | Md_L_DoneFailed=false;
      | }
  (junction 3) -> (junction 5) : {
      | IfVeSMSuSecRwLtStRclCmdSrv_Val_write=false;
      | Md_L_DoneOk=Md_L_DoneOkRaw;
      | Md_L_DoneFailed=Md_L_DoneFailedRaw;
      | }
  (junction 5) -> (junction 7)
  (junction 7) -> (junction 10)
  data: Left_Done input boolean; IfVeSMSuSecRwLtStRclCmdSrv_Val_write output boolean; IfVeSMSuSecRwLtStRclCmdSrv_Val_writeRaw input; Md_L_DoneOkRaw input; Md_L_DoneFailedRaw input; Md_L_DoneOk output boolean; Md_L_DoneFailed output boolean

== stateflow chart ModeAdjust/ModeAdjustRunnable_sys/ModeAdjust/RecvyL4s/Chart ==
  (default) -> (junction 3) : {failflg=0;}
  (junction 3) -> (junction 5) [order 1] : [!R2Lt_ini]
  (junction 5) -> (junction 9) [order 1] : [R2Lt_done]
  (junction 3) -> (junction 13) [order 2] : {R2Lt_En=false;}
  (junction 5) -> (junction 7) [order 2] : {R2Lt_En=true;}
  (junction 9) -> (junction 11) : {R2Lt_En=false;}
  (junction 7) -> (junction 13)
  (junction 11) -> (junction 7)
  (junction 13) -> (junction 237)
  (junction 237) -> (junction 244) [order 1] : [!HdUp_ini]
  (junction 244) -> (junction 234) [order 1] : [HdUp_Done]
  (junction 237) -> (junction 235) [order 2] : {HdUp_En =false;}
  (junction 244) -> (junction 246) [order 2] : {HdUp_En = true;}
  (junction 234) -> (junction 236) : {HdUp_En =false;}
  (junction 246) -> (junction 235)
  (junction 236) -> (junction 246)
  (junction 235) -> (junction 62)
  (junction 62) -> (junction 105) [order 1] : [!Step1_ini]
  (junction 105) -> (junction 107) [order 1] : [Step1done]
  (junction 62) -> (junction 68) [order 2] : {
      | StepEn_LgrstStep1=false;
      | }
  (junction 105) -> (junction 82) [order 2] : {StepEn_LgrstStep1=true;}
  (junction 107) -> (junction 109) : {StepEn_LgrstStep1=false;}
  (junction 82) -> (junction 68)
  (junction 109) -> (junction 82)
  (junction 68) -> (junction 143)
  (junction 143) -> (junction 142) [order 1] : [!Step2_ini]
  (junction 142) -> (junction 157) [order 1] : [downpos<=closedownpos2&&Ftpos>=FtposDelta]
  (junction 157) -> (junction 224) [order 1] : [Step1done&&Step3done]
  (junction 143) -> (junction 89) [order 2] : {
      | StepEn_LgrstStep2=false;
      | }
  (junction 142) -> (junction 154) [order 2]
  (junction 157) -> (junction 159) [order 2] : {
      | StepEn_LgrstStep2=false;
      | }
  (junction 224) -> (junction 228) : {failflg=1;}
  (junction 154) -> (junction 148) [order 1] : [downpos<closedownpos1&&Otpos>closeOtpos1]
  (junction 154) -> (junction 87) [order 2]
  (junction 148) -> (junction 150) : {StepEn_LgrstStep2 = false;}
  (junction 87) -> (junction 94) [order 1] : [Step2done]
  (junction 87) -> (junction 91) [order 2] : {
      | StepEn_LgrstStep2=true;
      | }
  (junction 94) -> (junction 96) : {
      | StepEn_LgrstStep2=false;
      | }
  (junction 91) -> (junction 89)
  (junction 96) -> (junction 91)
  (junction 150) -> (junction 96)
  (junction 159) -> (junction 150)
  (junction 228) -> (junction 159)
  (junction 89) -> (junction 101)
  (junction 101) -> (junction 113) [order 1] : [!Step3_ini]
  (junction 113) -> (junction 115) [order 1] : [Step3done||!Step1done]
  (junction 101) -> (junction 118) [order 2] : {
      | StepEn_LgrstStep3=false;
      | }
  (junction 113) -> (junction 258) [order 2]
  (junction 115) -> (junction 122) : {
      | StepEn_LgrstStep3=false;
      | }
  (junction 258) -> (junction 260) [order 1] : [downpos>closedownpos2]
  (junction 260) -> (junction 274) [order 1] : [Step2done]
  (junction 258) -> (junction 116) [order 2] : {
      | StepEn_LgrstStep3=true;
      | }
  (junction 260) -> (junction 262) [order 2] : {StepEn_LgrstStep3 = false;}
  (junction 274) -> (junction 276) : {
      | StepEn_LgrstStep3=true;
      | }
  (junction 116) -> (junction 118)
  (junction 262) -> (junction 116)
  (junction 276) -> (junction 262)
  (junction 122) -> (junction 276)
  (junction 118) -> (junction 182)
  (junction 182) -> (junction 178) [order 1] : [(Step1done&&Step2done&&Step3done)||failflg==1]
  (junction 178) -> (junction 252) [order 1] : [!HFwd_ini]
  (junction 252) -> (junction 173) [order 1] : [HdFwd_Done]
  (junction 182) -> (junction 181) [order 2]
  (junction 178) -> (junction 174) [order 2] : {HdFwd_En =false;}
  (junction 252) -> (junction 254) [order 2] : {HdFwd_En =true;}
  (junction 173) -> (junction 175) : {HdFwd_En =false;}
  (junction 254) -> (junction 174)
  (junction 175) -> (junction 254)
  (junction 174) -> (junction 176)
  (junction 176) -> (junction 181)
  (junction 181) -> (junction 165)
  data: R2Lt_ini input boolean; R2Lt_done input boolean; R2Lt_En output boolean; downpos input uint16; Otpos input uint16; Ftpos input uint16; closedownpos1 input uint16; closedownpos2 input uint16; closeOtpos1 input uint16; Step1done input boolean; Step2done input boolean; Step3done input boolean; Step1_ini input boolean; Step2_ini input boolean; Step3_ini input boolean; StepEn_LgrstStep1 output boolean; StepEn_LgrstStep2 output boolean; StepEn_LgrstStep3 output boolean; FtposDelta input uint16; HdFwd_Done input boolean; HdUp_Done input boolean; HdUp_En output boolean; HdFwd_En output boolean; OtposDelta input uint16; failflg output boolean; HdUp_ini input boolean; HFwd_ini input boolean

== stateflow chart ModeAdjust/ModeAdjustRunnable_sys/ModeAdjust/RecvyL4s/Chart1 ==
  (default) -> (junction 1)
  (junction 1) -> (junction 3) [order 1] : [Left_Done]
  (junction 1) -> (junction 7) [order 2] : {
      | IfVeSMSuSecRwLtStRclCmdSrv_Val_write=IfVeSMSuSecRwLtStRclCmdSrv_Val_writeRaw;
      | Md_L_DoneOk=false;
      | Md_L_DoneFailed=false;
      | }
  (junction 3) -> (junction 5) : {
      | IfVeSMSuSecRwLtStRclCmdSrv_Val_write=false;
      | Md_L_DoneOk=Md_L_DoneOkRaw;
      | Md_L_DoneFailed=Md_L_DoneFailedRaw;
      | }
  (junction 5) -> (junction 7)
  (junction 7) -> (junction 10)
  data: Left_Done input boolean; IfVeSMSuSecRwLtStRclCmdSrv_Val_write output boolean; IfVeSMSuSecRwLtStRclCmdSrv_Val_writeRaw input; Md_L_DoneOkRaw input; Md_L_DoneFailedRaw input; Md_L_DoneOk output boolean; Md_L_DoneFailed output boolean
